simulink model "powercontroller"  (R2015a)
settings: Solver=ode45  StartTime=0.0  StopTime=10.0  RelTol=1e-3
undefined symbols (not defined in the file): EngineSpeedPower, FuelConsTable, GasEmisTable
libraries: simulink x9, simulink_extras x1, powerlib_extras x1
settings Model: Creator=Elena  LastModifiedBy=Elena

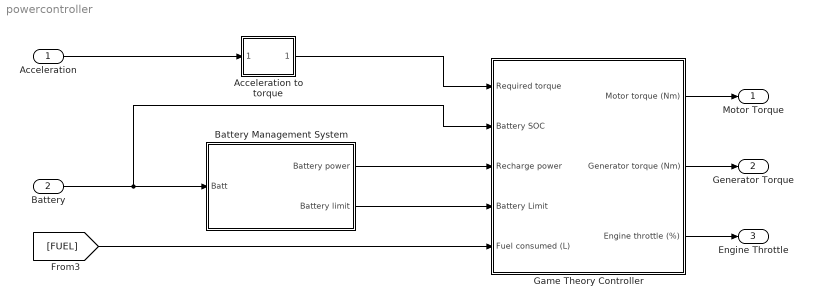
== system powercontroller ==
  Acceleration : Inport
  Battery : Inport  Port=2
  Acceleration to torque : Subsystem
      mask Display: plot([0;1800;2000;2500;3000;3500], [1;1;0.90*1;0.72*1;0.6*1;0.51*1])
  Battery Management System : Subsystem
      mask init:
      | [X1,X1m,X2,X2m,X3,X4,Y1,Y1m,Y2,Y2m,Y3,Y4,color1,color2]=spsdrivelogo;
      mask Display:
      | patch([X1 X1m],[Y1 Y1m],color1);
      | patch(X3,Y3,color2);
      | plot([X1 X1m X2 X2m X3 X4],[Y1 Y1m Y2 Y2m Y3 Y4]);
  Game Theory Controller : Subsystem
  Motor Torque : Outport
  Generator Torque : Outport  Port=2
  Engine Throttle : Outport  Port=3
  wires:
  Battery/1 -> Game Theory Controller/2(Battery SOC), Battery Management System/1(Batt)
  Battery Management System/2(Battery limit) -> Game Theory Controller/4(Battery Limit)
  Battery Management System/1(Battery power) -> Game Theory Controller/3(Recharge power)
  [FUEL] -> Game Theory Controller/5(Fuel consumed (L))
  Acceleration/1 -> Acceleration to torque/1(Acceleration)
  Acceleration to torque/1(torque) -> Game Theory Controller/1(Required torque)
  Game Theory Controller/3(Engine throttle (%)) -> Engine Throttle/1
  Game Theory Controller/2(Generator torque (Nm)) -> Generator Torque/1
  Game Theory Controller/1(Motor torque (Nm)) -> Motor Torque/1

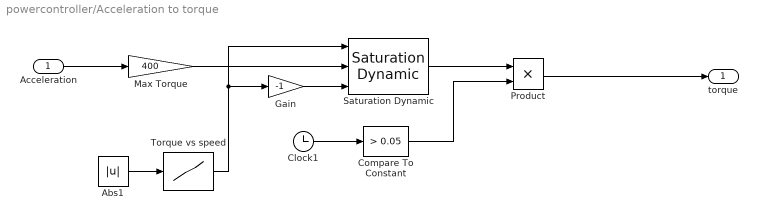
== system powercontroller/Acceleration to torque ==
  Acceleration : Inport
  Abs1 : Abs  SaturateOnIntegerOverflow=on
  Clock1 : Clock
  Compare To Constant : simulink/Logic and Bit Operations/Compare To Constant  relop=>  const=0.05  OutDataTypeStr=uint8  ZeroCross=off
  Gain : Gain  Gain=-1
  Max Torque : Gain  Gain=400
  Product : Product  RndMeth=Zero
  Saturation Dynamic : simulink/Discontinuities/Saturation Dynamic  OutMin=[]  OutMax=[]  OutDataTypeStr=Inherit: Same as second input  OutDataType=sfix(16)  OutScaling=2^-10  DoSatur=off
  Torque vs speed : Lookup  InputValues=[0 1200 2000 3000 4000 5000 6000]*pi/30  Table=[400 400 225 150 100 80 70]  LookUpMeth=Interpolation-Use End Values
  torque : Outport
  wires:
  ? -> Abs1/1
  Abs1/1 -> Torque vs speed/1
  Max Torque/1 -> Saturation Dynamic/2
  Torque vs speed/1 -> Gain/1, Saturation Dynamic/1
  Clock1/1 -> Compare To Constant/1
  Saturation Dynamic/1 -> Product/1
  Compare To Constant/1 -> Product/2
  Product/1 -> torque/1
  Gain/1 -> Saturation Dynamic/3
  Acceleration/1 -> Max Torque/1

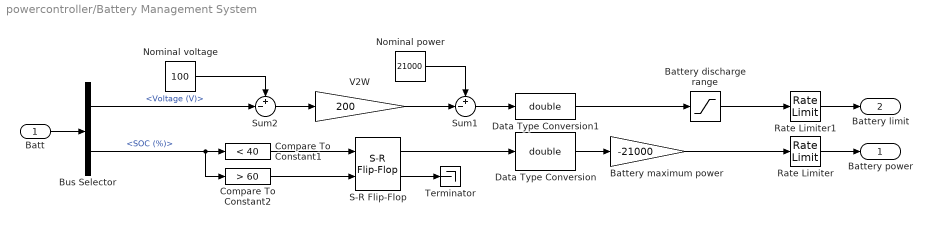
== system powercontroller/Battery Management System ==
  Batt : Inport
  Battery discharge range : Saturate  UpperLimit=21000  LowerLimit=0
  Battery maximum power : Gain  Gain=-21000
  Bus Selector : BusSelector  OutputSignals=Voltage (V),SOC (%)
  Compare To Constant1 : simulink/Logic and Bit Operations/Compare To Constant  relop=<  const=40  OutDataTypeStr=boolean
  Compare To Constant2 : simulink/Logic and Bit Operations/Compare To Constant  relop=>  const=60  OutDataTypeStr=boolean
  Data Type Conversion : DataTypeConversion  OutDataTypeStr=double  SampleTime=0
  Data Type Conversion1 : DataTypeConversion  OutDataTypeStr=double  SampleTime=0
  Nominal power : Constant  Value=21000
  Nominal voltage : Constant  Value=100
  Rate Limiter : RateLimiter  RisingSlewLimit=21000*2  FallingSlewLimit=-21000*2  SampleTimeMode=inherited
  Rate Limiter1 : RateLimiter  RisingSlewLimit=21000*10  FallingSlewLimit=-21000*10  SampleTimeMode=inherited
  S-R Flip-Flop : simulink_extras/Flip Flops/S-R Flip-Flop  initial_condition=0
  Sum1 : Sum  Inputs=+-|
  Sum2 : Sum  Inputs=+-|
  Terminator : Terminator
  V2W : Gain  Gain=200
  Battery power : Outport
  Battery limit : Outport  Port=2
  wires:
  Batt/1 -> Bus Selector/1
  Battery maximum power/1 -> Rate Limiter/1
  S-R Flip-Flop/2 -> Terminator/1
  Bus Selector/2 -> Compare To Constant1/1, Compare To Constant2/1  "<SOC (%)>"
  Data Type Conversion/1 -> Battery maximum power/1
  Compare To Constant1/1 -> S-R Flip-Flop/1
  Compare To Constant2/1 -> S-R Flip-Flop/2
  S-R Flip-Flop/1 -> Data Type Conversion/1
  Sum2/1 -> V2W/1
  V2W/1 -> Sum1/2
  Nominal power/1 -> Sum1/1
  Sum1/1 -> Data Type Conversion1/1
  Data Type Conversion1/1 -> Battery discharge range/1
  Battery discharge range/1 -> Rate Limiter1/1
  Bus Selector/1 -> Sum2/2  "<Voltage (V)>"
  Nominal voltage/1 -> Sum2/1
  Rate Limiter1/1 -> Battery limit/1
  Rate Limiter/1 -> Battery power/1

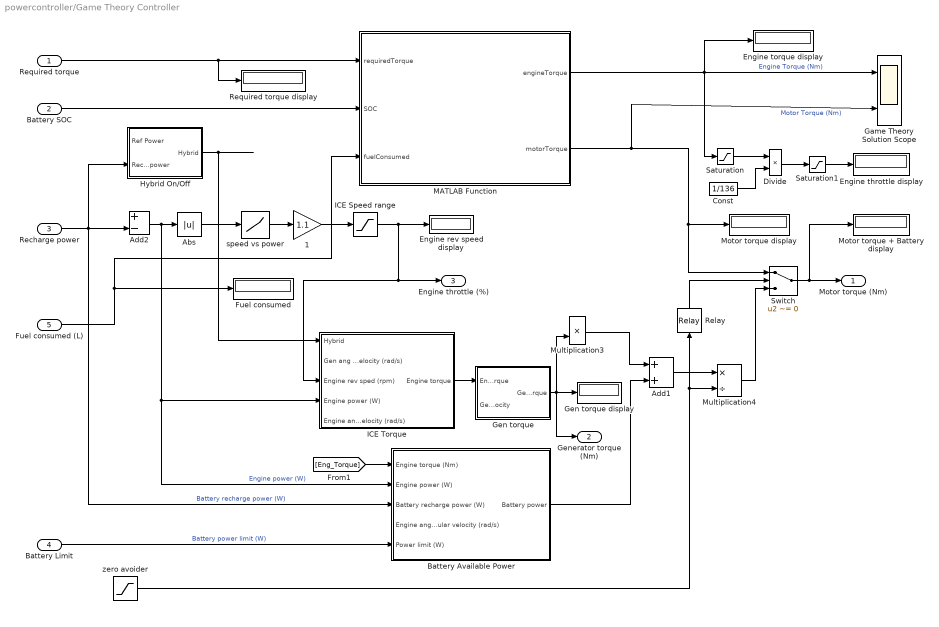
== system powercontroller/Game Theory Controller ==
  Required torque : Inport  OutDataTypeStr=double  PortDimensions=1
  Battery SOC : Inport  Port=2
  Recharge power : Inport  Port=3
  Battery Limit : Inport  Port=4
  Fuel consumed (L) : Inport  Port=5
  " 1" : Gain  Gain=1.1
  Abs : Abs
  Add1 : Sum
  Add2 : Sum  Inputs=+-
  Battery Available Power : Subsystem
  Const : Constant  Value=1/136
  Divide : Product  Inputs=**
  Engine rev speed display : Display
      settings: Decimation=100
  Engine throttle display : Display
      settings: Decimation=100
  Engine torque display : Display
      settings: Decimation=100
  Fuel consumed : Display
      settings: Decimation=100
  Game Theory Solution Scope : Scope  NumInputPorts=2
      settings: YMin=0~-225  YMax=140~275  SaveName=GameTheoryScope  Decimation=500
  Gen torque : Subsystem
  Gen torque display : Display
      settings: Decimation=100
  Hybrid On/Off : Subsystem
  ICE Speed range : Saturate  UpperLimit=5000  LowerLimit=750
  ICE Torque : Subsystem
  MATLAB Function : MATLAB Function  TreatAsAtomicUnit=on
  Motor torque + Battery display : Display
      settings: Decimation=100
  Motor torque display : Display
      settings: Decimation=100
  Multiplication3 : Product
  Multiplication4 : Product  Inputs=*/
  Relay : Relay  OnSwitchValue=200/30*pi  OffSwitchValue=100/30*pi  OnOutputValue=0  OffOutputValue=1
  Required torque display : Display
      settings: Decimation=100
  Saturation : Saturate  UpperLimit=136  LowerLimit=0
  Saturation1 : Saturate  UpperLimit=1  LowerLimit=0
  Switch : Switch  Criteria=u2 ~= 0
  speed vs power : Lookup  InputValues=EngineSpeedPower.power  Table=EngineSpeedPower.speed  SaturateOnIntegerOverflow=on
  zero avoider : Saturate  UpperLimit=inf  LowerLimit=1
  Motor torque (Nm) : Outport
  Generator torque (Nm) : Outport  Port=2
  Engine throttle (%) : Outport  Port=3
  wires:
  Required torque/1 -> Required torque display/1, MATLAB Function/1(requiredTorque)
  Battery SOC/1 -> MATLAB Function/2(SOC)
  ? -> Add2/1, Hybrid On/Off/1(Ref Power)
  Recharge power/1 -> Hybrid On/Off/2(Recharge power), Add2/2, Battery Available Power/3(Battery recharge power (W))  "Battery recharge power (W)"
  Add2/1 -> Abs/1, Battery Available Power/2(Engine power (W)), ICE Torque/4(Engine power (W))  "Engine power (W)"
  Abs/1 -> speed vs power/1
  speed vs power/1 -> " 1"/1
  " 1"/1 -> ICE Speed range/1
  Hybrid On/Off/1(Hybrid) -> ICE Torque/1(Hybrid)
  ? -> ICE Torque/5(Engine ang velocity (rad/s)), Battery Available Power/4(Engine angular velocity (rad/s))  "Engine angular velocity (rad/s)"
  ICE Torque/1(Engine torque) -> Gen torque/1(Engine torque)
  MATLAB Function/1(engineTorque) -> Engine torque display/1, Game Theory Solution Scope/1, Saturation/1  "Engine Torque (Nm)"
  Fuel consumed (L)/1 -> Fuel consumed/1, MATLAB Function/3(fuelConsumed)
  MATLAB Function/2(motorTorque) -> Game Theory Solution Scope/2, Switch/1, Motor torque display/1  "Motor Torque (Nm)"
  Gen torque/1(Gen torque) -> Multiplication3/2, Gen torque display/1, Generator torque (Nm)/1
  Saturation/1 -> Divide/1
  Const/1 -> Divide/2
  Divide/1 -> Saturation1/1
  Saturation1/1 -> Engine throttle display/1
  [Eng_Torque] -> Battery Available Power/1(Engine torque (Nm))
  Battery Limit/1 -> Battery Available Power/5(Power limit (W))  "Battery power limit (W)"
  ? -> zero avoider/1
  zero avoider/1 -> Multiplication4/2, Relay/1
  ? -> Multiplication3/1, Gen torque/2(Gen ang velocity), ICE Torque/2(Gen ang velocity (rad/s))  "Generator angular velocity (rad/s)"
  Multiplication3/1 -> Add1/1
  Battery Available Power/1(Battery power) -> Add1/2
  Add1/1 -> Multiplication4/1
  Multiplication4/1 -> Switch/3
  Switch/1 -> Motor torque (Nm)/1, Motor torque + Battery display/1
  Relay/1 -> Switch/2
  ICE Speed range/1 -> Engine throttle (%)/1, ICE Torque/3(Engine rev sped (rpm)), Engine rev speed display/1

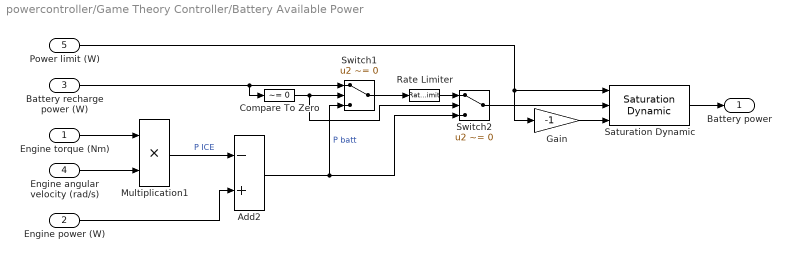
== system powercontroller/Game Theory Controller/Battery Available Power ==
  Engine torque (Nm) : Inport
  Engine power (W) : Inport  Port=2
  Battery recharge power (W) : Inport  Port=3
  Engine angular velocity (rad/s) : Inport  Port=4
  Power limit (W) : Inport  Port=5
  Add2 : Sum  Inputs=-+
  Compare To Zero : simulink/Logic and Bit Operations/Compare To Zero  relop=~=  OutDataTypeStr=boolean
  Gain : Gain  Gain=-1
  Multiplication1 : Product
  Rate Limiter : RateLimiter  RisingSlewLimit=21e3  FallingSlewLimit=-21e3  SampleTimeMode=inherited
  Saturation Dynamic : simulink/Discontinuities/Saturation Dynamic  OutMin=[]  OutMax=[]  OutDataTypeStr=Inherit: Same as second input  OutDataType=sfix(16)  OutScaling=2^-10  DoSatur=off
  Switch1 : Switch  Criteria=u2 ~= 0
  Switch2 : Switch  Criteria=u2 ~= 0
  Battery power : Outport
  wires:
  Engine angular velocity (rad/s)/1 -> Multiplication1/2
  Saturation Dynamic/1 -> Battery power/1
  Engine power (W)/1 -> Add2/2
  Power limit (W)/1 -> Gain/1, Saturation Dynamic/1
  Gain/1 -> Saturation Dynamic/3
  Engine torque (Nm)/1 -> Multiplication1/1
  Multiplication1/1 -> Add2/1  "P ICE"
  Battery recharge power (W)/1 -> Switch1/1, Compare To Zero/1
  Compare To Zero/1 -> Switch1/2, Switch2/2
  Add2/1 -> Switch1/3, Switch2/3  "P batt"
  Switch1/1 -> Rate Limiter/1
  Rate Limiter/1 -> Switch2/1
  Switch2/1 -> Saturation Dynamic/2

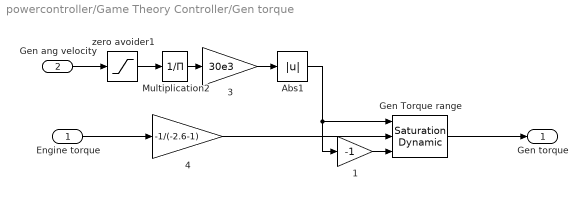
== system powercontroller/Game Theory Controller/Gen torque ==
  Engine torque : Inport
  Gen ang velocity : Inport  Port=2
  " 1" : Gain  Gain=-1
  " 3" : Gain  Gain=30e3
  " 4" : Gain  Gain=-1/(-2.6-1)
  Abs1 : Abs
  Gen Torque range : simulink/Discontinuities/Saturation Dynamic  OutMin=[]  OutMax=[]  OutDataTypeStr=Inherit: Same as second input  OutDataType=sfix(16)  OutScaling=2^-10  DoSatur=off
  Multiplication2 : Product  Inputs=/
  zero avoider1 : Saturate  UpperLimit=inf  LowerLimit=1
  Gen torque : Outport
  wires:
  Engine torque/1 -> " 4"/1
  Multiplication2/1 -> " 3"/1
  " 3"/1 -> Abs1/1
  Gen ang velocity/1 -> zero avoider1/1
  Abs1/1 -> Gen Torque range/1, " 1"/1
  " 1"/1 -> Gen Torque range/3
  " 4"/1 -> Gen Torque range/2
  Gen Torque range/1 -> Gen torque/1
  zero avoider1/1 -> Multiplication2/1

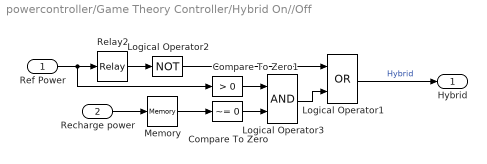
== system powercontroller/Game Theory Controller/Hybrid On//Off ==
  Ref Power : Inport
  Recharge power : Inport  Port=2
  Compare To Zero : simulink/Logic and Bit Operations/Compare To Zero  relop=~=  OutDataTypeStr=boolean
  Compare To Zero1 : simulink/Logic and Bit Operations/Compare To Zero  relop=>  OutDataTypeStr=boolean
  Logical Operator1 : Logic  Operator=OR  AllPortsSameDT=off  OutDataTypeStr=boolean
  Logical Operator2 : Logic  Operator=NOT  AllPortsSameDT=off  OutDataTypeStr=boolean
  Logical Operator3 : Logic  AllPortsSameDT=off  OutDataTypeStr=boolean
  Memory : Memory
  Relay2 : Relay  OnSwitchValue=12e3  OffSwitchValue=11e3  OnOutputValue=0  OffOutputValue=1
  Hybrid : Outport
  wires:
  Relay2/1 -> Logical Operator2/1
  Memory/1 -> Compare To Zero/1
  Logical Operator2/1 -> Logical Operator1/1
  Compare To Zero/1 -> Logical Operator3/2
  Logical Operator3/1 -> Logical Operator1/2
  Compare To Zero1/1 -> Logical Operator3/1
  Ref Power/1 -> Relay2/1, Compare To Zero1/1
  Recharge power/1 -> Memory/1
  Logical Operator1/1 -> Hybrid/1  "Hybrid"

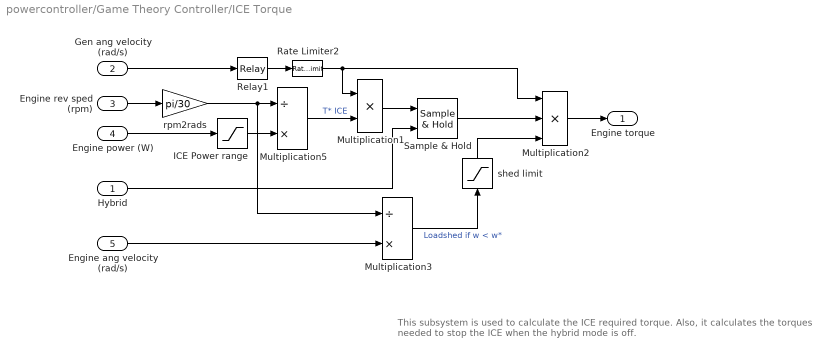
== system powercontroller/Game Theory Controller/ICE Torque ==
  note: This subsystem is used to calculate the ICE required torque.
      | Also, it calculates the torques needed to stop the ICE when the hybrid mode is off.
  Hybrid : Inport
  Gen ang velocity (rad/s) : Inport  Port=2
  Engine rev sped (rpm) : Inport  Port=3
  Engine power (W) : Inport  Port=4
  Engine ang velocity (rad/s) : Inport  Port=5
  ICE Power range : Saturate  UpperLimit=57e3  LowerLimit=-57e3
  Multiplication1 : Product
  Multiplication2 : Product  Inputs=3
  Multiplication3 : Product  Inputs=/*
  Multiplication5 : Product  Inputs=/*
  Rate Limiter2 : RateLimiter  RisingSlewLimit=10  FallingSlewLimit=-10
  Relay1 : Relay  OnSwitchValue=300  OffSwitchValue=200
  Sample & Hold : powerlib_extras/Control  Blocks/Sample & Hold  ic=0
  rpm2rads : Gain  Gain=pi/30
  shed limit : Saturate  UpperLimit=1  LowerLimit=0
  Engine torque : Outport
  wires:
  Relay1/1 -> Rate Limiter2/1
  Hybrid/1 -> Sample & Hold/2
  Engine power (W)/1 -> ICE Power range/1
  Engine rev sped (rpm)/1 -> rpm2rads/1
  Multiplication5/1 -> Multiplication1/2  "T* ICE"
  Multiplication1/1 -> Sample & Hold/1
  Multiplication2/1 -> Engine torque/1
  Rate Limiter2/1 -> Multiplication1/1, Multiplication2/1
  ICE Power range/1 -> Multiplication5/2
  rpm2rads/1 -> Multiplication5/1, Multiplication3/1
  Engine ang velocity (rad/s)/1 -> Multiplication3/2
  Multiplication3/1 -> shed limit/1  "Loadshed if w < w*"
  Sample & Hold/1 -> Multiplication2/2
  shed limit/1 -> Multiplication2/3
  Gen ang velocity (rad/s)/1 -> Relay1/1

== matlab function powercontroller/Game Theory Controller/MATLAB Function ==
  data: requiredTorque input double size=[1 1]; SOC input double; fuelConsumed input; engineTorque output double; motorTorque output double; FuelConsTable parameter; GasEmisTable parameter
function [engineTorque, motorTorque] = solveGame(requiredTorque, SOC, fuelConsumed, FuelConsTable, GasEmisTable)
%#codegen
    coder.extrinsic('int2str');
    coder.extrinsic('ismembertol');
    coder.extrinsic('knnsearch'); 
    coder.extrinsic('legend');
    coder.extrinsic('roundn');
    coder.extrinsic('solve');
 
  
   
    requiredTorqueR = 0;
    requiredTorqueR = roundn(requiredTorque,0);
       
    if requiredTorqueR > 0 && requiredTorqueR < 83     
       engineTorque = 0;
       motorTorque = requiredTorqueR;
    elseif requiredTorqueR < 0          
       engineTorque = 0;
       motorTorque = requiredTorqueR;
    elseif requiredTorqueR == 0          
       engineTorque = 0;
       motorTorque = 0;
    else  
        close all   
        motorSpeedCurve = [0, 1200, 2000, 3000, 4000, 5000, 6000];
        motorTorqueCurve = [400 399 225 150 100 80 70];
       
        SOC_deviation = abs(70 - SOC);       
        maxEngineTorque = 136;
        maxMotorTorque = 400;
        minMotorTorque = -400;
        minMotorTorqueRef = 0;
        minEngineTorqueRef = 83;
        minEngineTorque = 83;
        m = 7;
        e = 7;
        payoffMotor = zeros(m,e);
        payoffEngine = zeros(m,e);      
        if requiredTorque < 0
            maxMotorTorqueStrategy = 0;
            maxEngineTorqueStrategy = 0;
            minEngineTorqueStrategy = max(minEngineTorque, requiredTorque); 
            minMotorTorqueStrategy = max(minMotorTorque, requiredTorque);  
            strategyMot = linspace(minMotorTorqueStrategy, maxMotorTorqueStrategy, m);
            strategyEng = linspace(minEngineTorqueStrategy, maxEngineTorqueStrategy,e);
        else           
            maxEngineTorqueStrategy = min([requiredTorque maxEngineTorque]);
            maxMotorTorqueStrategy = min([requiredTorque maxMotorTorque]);    
            if minMotorTorqueRef > maxMotorTorqueStrategy
                strategyMot = zeros(1,m);
            else
                strategyMot = linspace(minMotorTorqueRef, maxMotorTorqueStrategy, m);
            end
            if minEngineTorqueRef > maxEngineTorqueStrategy
                strategyEng = zeros(1,e);
            else
                strategyEng = linspace(minEngineTorqueRef, maxEngineTorqueStrategy,e);
            end
        end          
          
        tmpTorque = repmat(strategyEng',1,m);
        totalTorque = zeros(m, e);
        for i = 1:m
            for j = 1:e
                totalTorque(i,j) = tmpTorque(i,j) + strategyMot(j);
            end
        end      
        
        % weights     
        wFuel = 3;
        wPower = 0.5;  
        wTank = 0.5;
        wDrDem = 0.5;
        wSOC = 1;
        wNOX = 65;
        wCO = 25;
        wHC = 45;
        motorSpeedRef = zeros(1,e);
       
        powerMotorKW = zeros(1,e);
        torqueDeviation = zeros(m,e);
        emissions = zeros(e,1);
        fuelConsRate = zeros(e,1);       
        power = zeros(e,1);
        for i = 1:m
            for j = 1:e
                tmpT = abs(FuelConsTable.torque - strategyEng(j));
                idxT = 0;                    
                % Power(W) = Torque (N.m) x Speed (RPM) / 9.5488
                % divide by 1000 for kW               
                motorSpeedRef(j) = interp1(motorTorqueCurve, motorSpeedCurve, abs(strategyMot(j)),'linear','extrap');
                powerMotorKW(j) = abs(strategyMot(j)) * motorSpeedRef(j) / 9.5488 / 1000;       
                tmpS = abs(FuelConsTable.speed - motorSpeedRef(j));
                idxS = 0;
                [~, idxS] = min(tmpS);
                [~, idxT] = min(tmpT);    
                fuelConsumedGPS = FuelConsTable.lookupTableFuel(idxT, idxS);
                HCEmissions = GasEmisTable.lookupTableHC(idxT, idxS);
                COEmissions = GasEmisTable.lookupTableCO(idxT, idxS);
                NOXEmissions = GasEmisTable.lookupTableNOX(idxT, idxS);   
                torqueDeviation(i,j) = requiredTorqueR - totalTorque(i,j);  
                emissions(j,1) = wHC*HCEmissions + wCO*COEmissions + wNOX*NOXEmissions;                
                payoffEngine(i,j) = wFuel*fuelConsumedGPS + wDrDem*abs(torqueDeviation(i,j)) + ...
                    wHC*HCEmissions + wCO*COEmissions + wNOX*NOXEmissions + ...
                    wTank*fuelConsumed;
                payoffMotor(i,j) = wDrDem*abs(torqueDeviation(i,j)) + wPower*powerMotorKW(j) + ...
                    wSOC*SOC_deviation;              
                fuelConsRate(j,1) = fuelConsumedGPS;      
                power(j,1) = powerMotorKW(j);                                
            end
        end
        [engineTorque, motorTorque] = solve(payoffEngine, payoffMotor, ...
        strategyEng, strategyMot, requiredTorqueR, torqueDeviation, fuelConsRate, fuelConsumed, emissions, power, m, e);            
    end
end
